simulink model "quadrupedRobot"  (R2020a)
settings: Solver=ode23tb  StartTime=0.0  StopTime=10  RelTol=1e-3
values from neighbouring files (symbols this model uses):
  BodyCenter_To_Arm = BodyLength*0.4    (= 0.24)    [Initial.m]
  BodyLength = 0.6    [Initial.m]
  BodyThick = 0.05    [Initial.m]
  BodyWidth = 0.25    [Initial.m]
  L1 = 0.1*L_total    (= 0.05)    [Initial.m]
  L2 = 0.4*L_total    (= 0.2)    [Initial.m]
  L3 = 0.5*L_total    (= 0.25)    [Initial.m]
  L_total = 0.5    [Initial.m]
  legX = 0.05    [Initial.m]
  legY = 0.05    [Initial.m]
  legZ = 0.05    [Initial.m]
  Mark = 1    [Initial.m]
  X = R_foot*cosd(0:0.2:90)    [Initial.m]
  X_FOOT = ([x_swing x_stance])/1000-S/2/2/1000    [Initial.m]
  Y = R_foot*sind(0:0.2:90)    [Initial.m]
  Y_FOOT = L1    (= 0.05)    [Initial.m]
  Z_FOOT = -L2-L3+Z_trajectory/1000+0.15    [Initial.m]
undefined symbols (not defined in the file or in its folder): Z
libraries: sm_lib x84, nesl_utility x27, Contact_Forces_Lib x5, simulink x1
(part 3 of 4)

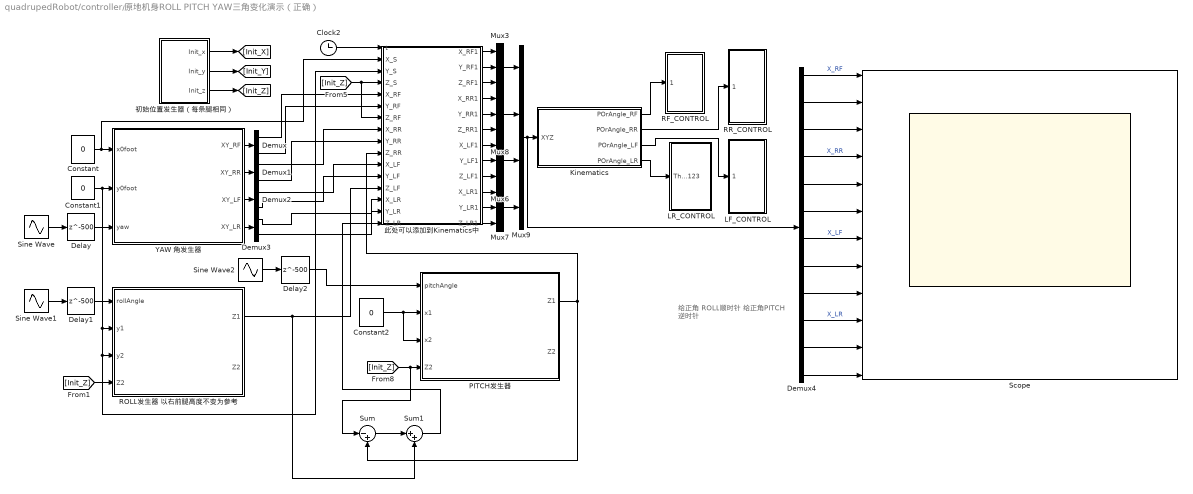
== system quadrupedRobot/controller/原地机身ROLL PITCH YAW三角变化演示（正确） ==
  note: 给正角 ROLL顺时针
      | 给正角PITCH 逆时针
  Clock2 : Clock
  Constant : Constant  Value=0
  Constant1 : Constant  Value=0
  Constant2 : Constant  Value=0
  Delay : Delay  DelayLength=500
  Delay1 : Delay  DelayLength=500
  Delay2 : Delay  DelayLength=500
  Demux{,1..3} (4 alike) : Demux  Outputs=2
  Demux4 : Demux  Outputs=12
  Kinematics : MATLAB Function  TreatAsAtomicUnit=on  mask{L1=L1, L2=L2, L3=L3, Mark=Mark}
  LF_CONTROL : Subsystem
  LR_CONTROL : Subsystem
  Mux{3,6..8} (4 alike) : Mux  Inputs=3
  Mux9 : Mux
  PITCH发生器 : MATLAB Function  TreatAsAtomicUnit=on
  RF_CONTROL : Subsystem
  ROLL发生器 以右前腿高度不变为参考 : MATLAB Function  TreatAsAtomicUnit=on
  RR_CONTROL : Subsystem
  Scope : Scope  NumInputPorts=12
  Sine Wave : Sin  Amplitude=8  Frequency=pi  SampleTime=0.001
  Sine Wave1 : Sin  Amplitude=8  Frequency=pi  SampleTime=0.001
  Sine Wave2 : Sin  Amplitude=8  Frequency=pi  SampleTime=0.001
  Sum : Sum  Inputs=|-+
  Sum1 : Sum  Inputs=|++
  YAW 角发生器 : MATLAB Function  TreatAsAtomicUnit=on
  初始位置发生器（每条腿相同） : Subsystem
  此处可以添加到Kinematics中 : Stateflow chart  TreatAsAtomicUnit=on
      settings: PortSchema="{\"entries\":[{\"content\":{\"sides\":[{\"content\":{\"connectorIds\":[\"In1\",\"In2\",\"In3\",\"In4\",\"In5\",\"In6\",\"In7\",\"In8\",\"In10\",\"In9\",\"In13\",\"In11\",\"In12\",\"In14\",\"In16\",\"In15\"]},\"type\":\"ConnectorPlacement.EquallySpacedRectSide\",\"uuid\":\"7e0be487-f0c2-4d3b-b1b4-d322333b651b\"},{\"content\":{\"connectorIds\":[\"Out11\",\"Out10\",\"Out9\",\"Out8\",\"Out6\",\"Out7\",\"Out3\",\"Out5\",\"Out4\",\"Out2\",\"Out12\",\"Out1\"],\"side\":\"RIGHT\"},\"type\":\"ConnectorPlacement.EquallySpacedRectSide\",\"uuid\":\"6febfd21-5bc4-4276-a755-f652306f84c9\"},{\"content\":{\"connectorIds\":[],\"side\":\"TOP\"},\"type\":\"ConnectorPlacement.EquallySpacedRectSide\",\"uuid\":\"b76ed853-f51f-41fe-9baf-83456c98e48b\"}]},\"type\":\"ConnectorPlacement.EquallySpacedConnector\",\"uuid\":\"3d522894-fd20-4e97-8ed2-383d7ec977f7\"}],\"packageUris\":[\"http://schema.mathworks.com/mf0/Connector/19700101\"],\"version\":\"1.0\"}"
  wires:
  Delay/1 -> YAW 角发生器/3(yaw)
  Demux3/2 -> 此处可以添加到Kinematics中/16(Y_LR)
  Demux3/1 -> 此处可以添加到Kinematics中/14(X_LR)
  YAW 角发生器/4(XY_LR) -> Demux3/1
  Demux2/2 -> 此处可以添加到Kinematics中/11(Y_LF)
  Demux2/1 -> 此处可以添加到Kinematics中/13(X_LF)
  YAW 角发生器/3(XY_LF) -> Demux2/1
  Demux1/1 -> 此处可以添加到Kinematics中/8(X_RR)
  YAW 角发生器/2(XY_RR) -> Demux1/1
  Demux/2 -> 此处可以添加到Kinematics中/6(Y_RF)
  Demux/1 -> 此处可以添加到Kinematics中/5(X_RF)
  YAW 角发生器/1(XY_RF) -> Demux/1
  Sine Wave/1 -> Delay/1
  初始位置发生器（每条腿相同）/1(Init_x) -> [Init_X]
  初始位置发生器（每条腿相同）/2(Init_y) -> [Init_Y]
  初始位置发生器（每条腿相同）/3(Init_z) -> [Init_Z]
  Constant/1 -> 此处可以添加到Kinematics中/2(X_S), YAW 角发生器/1(x0foot)
  [Init_Z] -> 此处可以添加到Kinematics中/7(Z_RF), 此处可以添加到Kinematics中/4(Z_S)
  Clock2/1 -> 此处可以添加到Kinematics中/1(t)
  此处可以添加到Kinematics中/11(X_RF1) -> Mux3/1
  此处可以添加到Kinematics中/10(Y_RF1) -> Mux3/2
  此处可以添加到Kinematics中/9(Z_RF1) -> Mux3/3
  此处可以添加到Kinematics中/8(X_RR1) -> Mux8/1
  此处可以添加到Kinematics中/6(Y_RR1) -> Mux8/2
  此处可以添加到Kinematics中/7(Z_RR1) -> Mux8/3
  此处可以添加到Kinematics中/3(X_LF1) -> Mux6/1
  此处可以添加到Kinematics中/5(Y_LF1) -> Mux6/2
  此处可以添加到Kinematics中/4(Z_LF1) -> Mux6/3
  此处可以添加到Kinematics中/2(X_LR1) -> Mux7/1
  此处可以添加到Kinematics中/12(Y_LR1) -> Mux7/2
  此处可以添加到Kinematics中/1(Z_LR1) -> Mux7/3
  Mux3/1 -> Mux9/1
  Mux8/1 -> Mux9/2
  Mux6/1 -> Mux9/3
  Mux7/1 -> Mux9/4
  Mux9/1 -> Demux4/1, Kinematics/1(XYZ)
  Kinematics/1(POrAngle_RF) -> RF_CONTROL/1(Theta123)
  Kinematics/2(POrAngle_RR) -> RR_CONTROL/1(Theta123)
  Kinematics/3(POrAngle_LF) -> LF_CONTROL/1(Theta123)
  Kinematics/4(POrAngle_LR) -> LR_CONTROL/1(Theta123)
  Sine Wave1/1 -> Delay1/1
  Delay1/1 -> ROLL发生器 以右前腿高度不变为参考/1(rollAngle)
  [Init_Z] -> ROLL发生器 以右前腿高度不变为参考/4("Z2 ")
  Constant1/1 -> ROLL发生器 以右前腿高度不变为参考/3(y2), 此处可以添加到Kinematics中/3(Y_S), ROLL发生器 以右前腿高度不变为参考/2(y1), YAW 角发生器/2(y0foot)
  ROLL发生器 以右前腿高度不变为参考/1(Z1) -> Sum1/2, 此处可以添加到Kinematics中/12(Z_LF)
  Constant2/1 -> PITCH发生器/2(x1), PITCH发生器/3(x2)
  PITCH发生器/1(Z1) -> Sum/2, 此处可以添加到Kinematics中/9(Z_RR)
  Sum/1 -> Sum1/1
  [Init_Z] -> Sum/1, PITCH发生器/4("Z2 ")
  Sum1/1 -> 此处可以添加到Kinematics中/15(Z_LR)
  Sine Wave2/1 -> Delay2/1
  Delay2/1 -> PITCH发生器/1(pitchAngle)
  Demux1/2 -> 此处可以添加到Kinematics中/10(Y_RR)
  Demux4/1 -> Scope/1  "X_RF"
  Demux4/2 -> Scope/2
  Demux4/3 -> Scope/3
  Demux4/4 -> Scope/4  "X_RR"
  Demux4/5 -> Scope/5
  Demux4/6 -> Scope/6
  Demux4/7 -> Scope/7  "X_LF"
  Demux4/8 -> Scope/8
  Demux4/9 -> Scope/9
  Demux4/10 -> Scope/10  "X_LR"
  Demux4/11 -> Scope/11
  Demux4/12 -> Scope/12

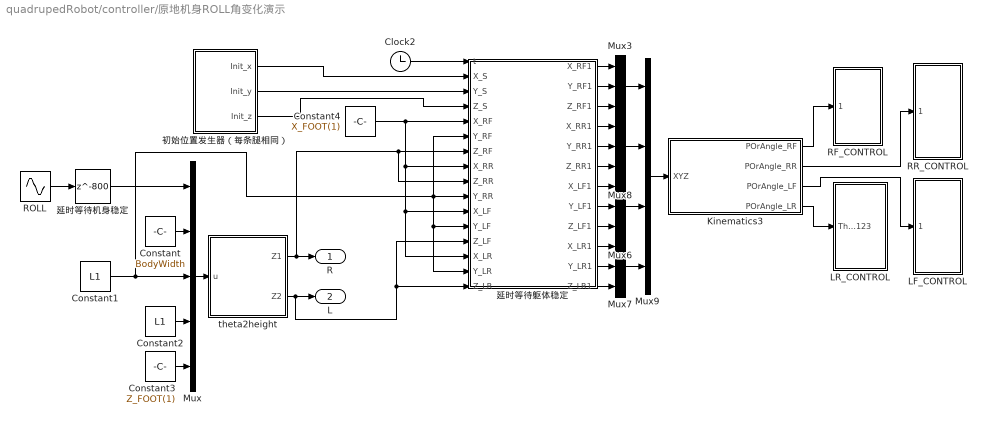
== system quadrupedRobot/controller/原地机身ROLL角变化演示 ==
  Clock2 : Clock
  Constant : Constant  Value=BodyWidth
  Constant1 : Constant  Value=L1
  Constant2 : Constant  Value=L1
  Constant3 : Constant  Value=Z_FOOT(1)
  Constant4 : Constant  Value=X_FOOT(1)
  Kinematics3 : MATLAB Function  TreatAsAtomicUnit=on  mask{L1=L1, L2=L2, L3=L3, Mark=Mark}
  LF_CONTROL : Subsystem
  LR_CONTROL : Subsystem
  Mux : Mux  Inputs=5
  Mux{3,6..8} (4 alike) : Mux  Inputs=3
  Mux9 : Mux
  RF_CONTROL : Subsystem
  ROLL : Sin  Amplitude=5  Frequency=3*pi  SampleTime=0.001
  RR_CONTROL : Subsystem
  theta2height : MATLAB Function  TreatAsAtomicUnit=on
  初始位置发生器（每条腿相同） : Subsystem
  延时等待机身稳定 : Delay  DelayLength=800
  延时等待躯体稳定 : Stateflow chart  TreatAsAtomicUnit=on
      settings: PortSchema="{\"entries\":[{\"content\":{\"sides\":[{\"content\":{\"connectorIds\":[\"In1\",\"In2\",\"In3\",\"In4\",\"In5\",\"In6\",\"In7\",\"In8\",\"In9\",\"In10\",\"In13\",\"In11\",\"In12\",\"In14\",\"In16\",\"In15\"]},\"type\":\"ConnectorPlacement.EquallySpacedRectSide\",\"uuid\":\"7e0be487-f0c2-4d3b-b1b4-d322333b651b\"},{\"content\":{\"connectorIds\":[\"Out11\",\"Out10\",\"Out9\",\"Out8\",\"Out6\",\"Out7\",\"Out3\",\"Out5\",\"Out4\",\"Out2\",\"Out12\",\"Out1\"],\"side\":\"RIGHT\"},\"type\":\"ConnectorPlacement.EquallySpacedRectSide\",\"uuid\":\"6febfd21-5bc4-4276-a755-f652306f84c9\"},{\"content\":{\"connectorIds\":[],\"side\":\"TOP\"},\"type\":\"ConnectorPlacement.EquallySpacedRectSide\",\"uuid\":\"b76ed853-f51f-41fe-9baf-83456c98e48b\"}]},\"type\":\"ConnectorPlacement.EquallySpacedConnector\",\"uuid\":\"3d522894-fd20-4e97-8ed2-383d7ec977f7\"}],\"packageUris\":[\"http://schema.mathworks.com/mf0/Connector/19700101\"],\"version\":\"1.0\"}"
  R : Outport
  L : Outport  Port=2
  wires:
  theta2height/2(Z2) -> 延时等待躯体稳定/12(Z_LF), 延时等待躯体稳定/15(Z_LR), L/1
  Mux/1 -> theta2height/1(u)
  ROLL/1 -> 延时等待机身稳定/1
  theta2height/1(Z1) -> 延时等待躯体稳定/9(Z_RR), 延时等待躯体稳定/7(Z_RF), R/1
  Kinematics3/3(POrAngle_LF) -> LF_CONTROL/1(Theta123)
  Kinematics3/2(POrAngle_RR) -> RR_CONTROL/1(Theta123)
  Mux8/1 -> Mux9/2
  延时等待躯体稳定/5(Y_LF1) -> Mux6/2
  Mux9/1 -> Kinematics3/1(XYZ)
  延时等待躯体稳定/1(Z_LR1) -> Mux7/3
  延时等待躯体稳定/11(X_RF1) -> Mux3/1
  延时等待躯体稳定/3(X_LF1) -> Mux6/1
  延时等待躯体稳定/6(Y_RR1) -> Mux8/2
  延时等待躯体稳定/2(X_LR1) -> Mux7/1
  延时等待躯体稳定/10(Y_RF1) -> Mux3/2
  延时等待躯体稳定/12(Y_LR1) -> Mux7/2
  Mux3/1 -> Mux9/1
  延时等待躯体稳定/9(Z_RF1) -> Mux3/3
  延时等待躯体稳定/7(Z_RR1) -> Mux8/3
  延时等待躯体稳定/4(Z_LF1) -> Mux6/3
  Kinematics3/1(POrAngle_RF) -> RF_CONTROL/1(Theta123)
  延时等待躯体稳定/8(X_RR1) -> Mux8/1
  初始位置发生器（每条腿相同）/2(Init_y) -> 延时等待躯体稳定/3(Y_S)
  Mux6/1 -> Mux9/3
  初始位置发生器（每条腿相同）/3(Init_z) -> 延时等待躯体稳定/4(Z_S)
  Clock2/1 -> 延时等待躯体稳定/1(t)
  Mux7/1 -> Mux9/4
  Kinematics3/4(POrAngle_LR) -> LR_CONTROL/1(Theta123)
  初始位置发生器（每条腿相同）/1(Init_x) -> 延时等待躯体稳定/2(X_S)
  Constant/1 -> Mux/2
  Constant1/1 -> Mux/3, 延时等待躯体稳定/6(Y_RF), 延时等待躯体稳定/11(Y_LF), 延时等待躯体稳定/16(Y_LR), 延时等待躯体稳定/10(Y_RR)
  Constant2/1 -> Mux/4
  Constant3/1 -> Mux/5
  Constant4/1 -> 延时等待躯体稳定/14(X_LR), 延时等待躯体稳定/13(X_LF), 延时等待躯体稳定/8(X_RR), 延时等待躯体稳定/5(X_RF)
  延时等待机身稳定/1 -> Mux/1

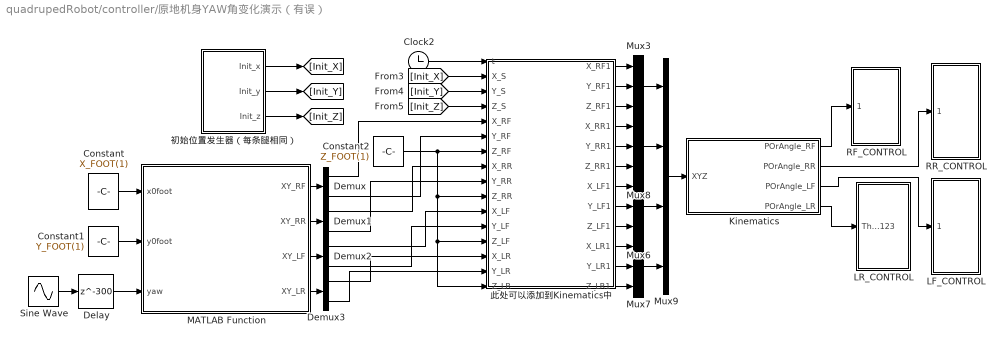
== system quadrupedRobot/controller/原地机身YAW角变化演示（有误） ==
  Clock2 : Clock
  Constant : Constant  Value=X_FOOT(1)
  Constant1 : Constant  Value=Y_FOOT(1)
  Constant2 : Constant  Value=Z_FOOT(1)
  Delay : Delay  DelayLength=300
  Demux{,1..3} (4 alike) : Demux  Outputs=2
  Kinematics : MATLAB Function  TreatAsAtomicUnit=on  mask{L1=L1, L2=L2, L3=L3, Mark=Mark}
  LF_CONTROL : Subsystem
  LR_CONTROL : Subsystem
  MATLAB Function : MATLAB Function  TreatAsAtomicUnit=on
  Mux{3,6..8} (4 alike) : Mux  Inputs=3
  Mux9 : Mux
  RF_CONTROL : Subsystem
  RR_CONTROL : Subsystem
  Sine Wave : Sin  Amplitude=10  Frequency=2*pi  SampleTime=0.001
  初始位置发生器（每条腿相同） : Subsystem
  此处可以添加到Kinematics中 : Stateflow chart  TreatAsAtomicUnit=on
      settings: PortSchema="{\"entries\":[{\"content\":{\"sides\":[{\"content\":{\"connectorIds\":[\"In1\",\"In2\",\"In3\",\"In4\",\"In5\",\"In6\",\"In7\",\"In8\",\"In10\",\"In9\",\"In13\",\"In11\",\"In12\",\"In14\",\"In16\",\"In15\"]},\"type\":\"ConnectorPlacement.EquallySpacedRectSide\",\"uuid\":\"7e0be487-f0c2-4d3b-b1b4-d322333b651b\"},{\"content\":{\"connectorIds\":[\"Out11\",\"Out10\",\"Out9\",\"Out8\",\"Out6\",\"Out7\",\"Out3\",\"Out5\",\"Out4\",\"Out2\",\"Out12\",\"Out1\"],\"side\":\"RIGHT\"},\"type\":\"ConnectorPlacement.EquallySpacedRectSide\",\"uuid\":\"6febfd21-5bc4-4276-a755-f652306f84c9\"},{\"content\":{\"connectorIds\":[],\"side\":\"TOP\"},\"type\":\"ConnectorPlacement.EquallySpacedRectSide\",\"uuid\":\"b76ed853-f51f-41fe-9baf-83456c98e48b\"}]},\"type\":\"ConnectorPlacement.EquallySpacedConnector\",\"uuid\":\"3d522894-fd20-4e97-8ed2-383d7ec977f7\"}],\"packageUris\":[\"http://schema.mathworks.com/mf0/Connector/19700101\"],\"version\":\"1.0\"}"
  wires:
  Kinematics/4(POrAngle_LR) -> LR_CONTROL/1(Theta123)
  Kinematics/3(POrAngle_LF) -> LF_CONTROL/1(Theta123)
  Kinematics/2(POrAngle_RR) -> RR_CONTROL/1(Theta123)
  Kinematics/1(POrAngle_RF) -> RF_CONTROL/1(Theta123)
  Mux9/1 -> Kinematics/1(XYZ)
  Mux7/1 -> Mux9/4
  Mux6/1 -> Mux9/3
  Mux8/1 -> Mux9/2
  Mux3/1 -> Mux9/1
  此处可以添加到Kinematics中/1(Z_LR1) -> Mux7/3
  此处可以添加到Kinematics中/12(Y_LR1) -> Mux7/2
  此处可以添加到Kinematics中/2(X_LR1) -> Mux7/1
  此处可以添加到Kinematics中/4(Z_LF1) -> Mux6/3
  此处可以添加到Kinematics中/5(Y_LF1) -> Mux6/2
  此处可以添加到Kinematics中/3(X_LF1) -> Mux6/1
  此处可以添加到Kinematics中/7(Z_RR1) -> Mux8/3
  此处可以添加到Kinematics中/6(Y_RR1) -> Mux8/2
  此处可以添加到Kinematics中/8(X_RR1) -> Mux8/1
  此处可以添加到Kinematics中/9(Z_RF1) -> Mux3/3
  此处可以添加到Kinematics中/10(Y_RF1) -> Mux3/2
  此处可以添加到Kinematics中/11(X_RF1) -> Mux3/1
  Clock2/1 -> 此处可以添加到Kinematics中/1(t)
  [Init_Z] -> 此处可以添加到Kinematics中/4(Z_S)
  [Init_Y] -> 此处可以添加到Kinematics中/3(Y_S)
  [Init_X] -> 此处可以添加到Kinematics中/2(X_S)
  初始位置发生器（每条腿相同）/3(Init_z) -> [Init_Z]
  初始位置发生器（每条腿相同）/2(Init_y) -> [Init_Y]
  初始位置发生器（每条腿相同）/1(Init_x) -> [Init_X]
  ? -> ?
  Constant/1 -> MATLAB Function/1(x0foot)
  Constant1/1 -> MATLAB Function/2(y0foot)
  Sine Wave/1 -> Delay/1
  Constant2/1 -> 此处可以添加到Kinematics中/15(Z_LR), 此处可以添加到Kinematics中/12(Z_LF), 此处可以添加到Kinematics中/9(Z_RR), 此处可以添加到Kinematics中/7(Z_RF)
  MATLAB Function/1(XY_RF) -> Demux/1
  Demux/1 -> 此处可以添加到Kinematics中/5(X_RF)
  Demux/2 -> 此处可以添加到Kinematics中/6(Y_RF)
  MATLAB Function/2(XY_RR) -> Demux1/1
  Demux1/1 -> 此处可以添加到Kinematics中/8(X_RR)
  Demux1/2 -> 此处可以添加到Kinematics中/10(Y_RR)
  MATLAB Function/3(XY_LF) -> Demux2/1
  Demux2/1 -> 此处可以添加到Kinematics中/13(X_LF)
  Demux2/2 -> 此处可以添加到Kinematics中/11(Y_LF)
  MATLAB Function/4(XY_LR) -> Demux3/1
  Demux3/1 -> 此处可以添加到Kinematics中/14(X_LR)
  Demux3/2 -> 此处可以添加到Kinematics中/16(Y_LR)
  Delay/1 -> MATLAB Function/3(yaw)

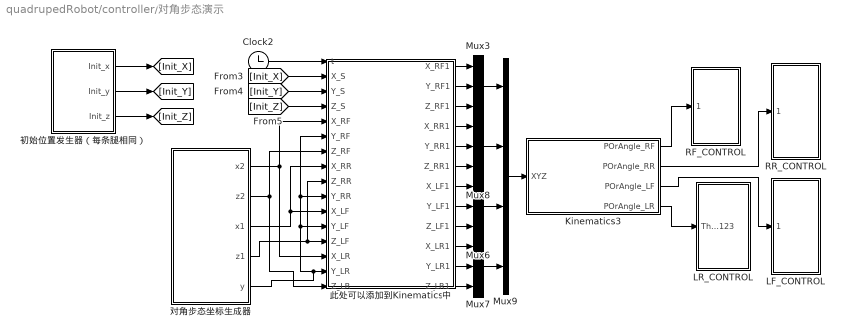
== system quadrupedRobot/controller/对角步态演示 ==
  Clock2 : Clock
  Kinematics3 : MATLAB Function  TreatAsAtomicUnit=on  mask{L1=L1, L2=L2, L3=L3, Mark=Mark}
  LF_CONTROL : Subsystem
  LR_CONTROL : Subsystem
  Mux{3,6..8} (4 alike) : Mux  Inputs=3
  Mux9 : Mux
  RF_CONTROL : Subsystem
  RR_CONTROL : Subsystem
  初始位置发生器（每条腿相同） : Subsystem
  对角步态坐标生成器 : Subsystem
  此处可以添加到Kinematics中 : Stateflow chart  TreatAsAtomicUnit=on
      settings: PortSchema="{\"entries\":[{\"content\":{\"sides\":[{\"content\":{\"connectorIds\":[\"In1\",\"In2\",\"In3\",\"In4\",\"In5\",\"In6\",\"In7\",\"In8\",\"In9\",\"In10\",\"In13\",\"In11\",\"In12\",\"In14\",\"In16\",\"In15\"]},\"type\":\"ConnectorPlacement.EquallySpacedRectSide\",\"uuid\":\"7e0be487-f0c2-4d3b-b1b4-d322333b651b\"},{\"content\":{\"connectorIds\":[\"Out11\",\"Out10\",\"Out9\",\"Out8\",\"Out6\",\"Out7\",\"Out3\",\"Out5\",\"Out4\",\"Out2\",\"Out12\",\"Out1\"],\"side\":\"RIGHT\"},\"type\":\"ConnectorPlacement.EquallySpacedRectSide\",\"uuid\":\"6febfd21-5bc4-4276-a755-f652306f84c9\"},{\"content\":{\"connectorIds\":[],\"side\":\"TOP\"},\"type\":\"ConnectorPlacement.EquallySpacedRectSide\",\"uuid\":\"b76ed853-f51f-41fe-9baf-83456c98e48b\"}]},\"type\":\"ConnectorPlacement.EquallySpacedConnector\",\"uuid\":\"3d522894-fd20-4e97-8ed2-383d7ec977f7\"}],\"packageUris\":[\"http://schema.mathworks.com/mf0/Connector/19700101\"],\"version\":\"1.0\"}"
  wires:
  ? -> ?
  初始位置发生器（每条腿相同）/1(Init_x) -> [Init_X]
  初始位置发生器（每条腿相同）/2(Init_y) -> [Init_Y]
  初始位置发生器（每条腿相同）/3(Init_z) -> [Init_Z]
  [Init_X] -> 此处可以添加到Kinematics中/2(X_S)
  [Init_Y] -> 此处可以添加到Kinematics中/3(Y_S)
  [Init_Z] -> 此处可以添加到Kinematics中/4(Z_S)
  Clock2/1 -> 此处可以添加到Kinematics中/1(t)
  此处可以添加到Kinematics中/11(X_RF1) -> Mux3/1
  此处可以添加到Kinematics中/10(Y_RF1) -> Mux3/2
  此处可以添加到Kinematics中/9(Z_RF1) -> Mux3/3
  此处可以添加到Kinematics中/8(X_RR1) -> Mux8/1
  此处可以添加到Kinematics中/6(Y_RR1) -> Mux8/2
  此处可以添加到Kinematics中/7(Z_RR1) -> Mux8/3
  此处可以添加到Kinematics中/3(X_LF1) -> Mux6/1
  此处可以添加到Kinematics中/5(Y_LF1) -> Mux6/2
  此处可以添加到Kinematics中/4(Z_LF1) -> Mux6/3
  此处可以添加到Kinematics中/2(X_LR1) -> Mux7/1
  此处可以添加到Kinematics中/12(Y_LR1) -> Mux7/2
  此处可以添加到Kinematics中/1(Z_LR1) -> Mux7/3
  Mux3/1 -> Mux9/1
  Mux8/1 -> Mux9/2
  Mux6/1 -> Mux9/3
  Mux7/1 -> Mux9/4
  Mux9/1 -> Kinematics3/1(XYZ)
  Kinematics3/1(POrAngle_RF) -> RF_CONTROL/1(Theta123)
  Kinematics3/2(POrAngle_RR) -> RR_CONTROL/1(Theta123)
  Kinematics3/3(POrAngle_LF) -> LF_CONTROL/1(Theta123)
  Kinematics3/4(POrAngle_LR) -> LR_CONTROL/1(Theta123)
  对角步态坐标生成器/5(y) -> 此处可以添加到Kinematics中/11(Y_LF), 此处可以添加到Kinematics中/6(Y_RF), 此处可以添加到Kinematics中/10(Y_RR), 此处可以添加到Kinematics中/16(Y_LR)
  对角步态坐标生成器/1(x2) -> 此处可以添加到Kinematics中/14(X_LR), 此处可以添加到Kinematics中/5(X_RF)
  对角步态坐标生成器/2(z2) -> 此处可以添加到Kinematics中/7(Z_RF), 此处可以添加到Kinematics中/15(Z_LR)
  对角步态坐标生成器/3(x1) -> 此处可以添加到Kinematics中/13(X_LF), 此处可以添加到Kinematics中/8(X_RR)
  对角步态坐标生成器/4(z1) -> 此处可以添加到Kinematics中/9(Z_RR), 此处可以添加到Kinematics中/12(Z_LF)

== system quadrupedRobot/Robot/LF/Subsystem ==
  shoulderJoint : Inport
  R1 : sm_lib/Joints/Revolute Joint  JointMode=Normal  SenseConstraintForce=off  SenseConstraintForceX=off  SenseConstraintForceY=off  SenseConstraintForceZ=off  SenseConstraintTorque=off  SenseConstraintTorqueX=off  SenseConstraintTorqueY=off  SenseConstraintTorqueZ=off  SenseTotalForce=off  SenseTotalForceX=off  SenseTotalForceY=off  SenseTotalForceZ=off  SenseTotalTorque=off  SenseTotalTorqueX=off  SenseTotalTorqueY=off  SenseTotalTorqueZ=off  CompositeWrenchDir=FollowerOnBase  CompositeWrenchFrame=BaseFrame  EquilibriumPosition=0  EquilibriumPositionUnits=deg  SpringStiffness=0  SpringStiffnessUnits=N*m/deg  DampingCoefficient=0  DampingCoefficientUnits=N*m/(deg/s)  TorqueActuationMode=ComputedTorque  MotionActuationMode=InputMotion  SensePosition=off  SenseVelocity=off  SenseAcceleration=off  SenseTorqueForce=off  SenseLowerLimitTorqueForce=off  SenseUpperLimitTorqueForce=off  LowerLimitSpecify=off  LowerLimitBound=-90  LowerLimitBoundUnits=deg  LowerLimitStiffness=1e4  LowerLimitStiffnessUnits=N*m/deg  LowerLimitDamping=10  LowerLimitDampingUnits=N*m/(deg/s)  LowerLimitTransitionRegionWidth=0.1  LowerLimitTransitionRegionWidthUnits=deg  UpperLimitSpecify=off  UpperLimitBound=90  UpperLimitBoundUnits=deg  UpperLimitStiffness=1e4  UpperLimitStiffnessUnits=N*m/deg  UpperLimitDamping=10  UpperLimitDampingUnits=N*m/(deg/s)  UpperLimitTransitionRegionWidth=0.1  UpperLimitTransitionRegionWidthUnits=deg  PositionTargetSpecify=on  PositionTargetPriority=High  PositionTargetValue=0  PositionTargetValueUnits=deg  VelocityTargetSpecify=off  VelocityTargetPriority=High  VelocityTargetValue=0  VelocityTargetValueUnits=deg/s
  Rigid Transform8 : sm_lib/Frames and Transforms/Rigid Transform  TranslationMethod=None  TranslationStandardOffset=0  TranslationLengthUnit=m  TranslationStandardAxis=+Z  TranslationCartesianOffset=[0 0 0]  TranslationROffset=0  TranslationROffsetUnits=m  TranslationZOffset=0  TranslationZOffsetUnits=m  TranslationThetaOffset=0  TranslationThetaOffsetUnits=deg  RotationMethod=StandardAxis  RotationAngleUnits=deg  RotationStandardAxis=+Y  RotationAngle=90  RotationArbitraryAxis=[0 0 1]  FollAlignAxisA=+X  BaseAlignAxisA=+Y  FollAlignAxisB=+Y  BaseAlignAxisB=+Z  RotationSequenceAxes=FollowerAxes  RotationSequence=XYX  RotationSequenceAngles=[0 0 0]  RotationSequenceAnglesUnits=deg  RotationMatrix=[1 0 0; 0 1 0; 0 0 1]
  Rigid Transform9 : sm_lib/Frames and Transforms/Rigid Transform  TranslationMethod=None  TranslationStandardOffset=0  TranslationLengthUnit=m  TranslationStandardAxis=+Z  TranslationCartesianOffset=[0 0 0]  TranslationROffset=0  TranslationROffsetUnits=m  TranslationZOffset=0  TranslationZOffsetUnits=m  TranslationThetaOffset=0  TranslationThetaOffsetUnits=deg  RotationMethod=StandardAxis  RotationAngleUnits=deg  RotationStandardAxis=+Y  RotationAngle=90  RotationArbitraryAxis=[0 0 1]  FollAlignAxisA=+X  BaseAlignAxisA=+Y  FollAlignAxisB=+Y  BaseAlignAxisB=+Z  RotationSequenceAxes=FollowerAxes  RotationSequence=XYX  RotationSequenceAngles=[0 0 0]  RotationSequenceAnglesUnits=deg  RotationMatrix=[1 0 0; 0 1 0; 0 0 1]
  Simulink-PS Converter4 : nesl_utility/Simulink-PS Converter  PhysicalDomain=network_engine_domain  SubClassName=ps_input  LeftPortType=input  RightPortType=output  PseudoPeriodic=off  Frequencies=[]  NoiseDistribution=none  NoiseParameters=[]  Unit=1  AffineConversion=off  FilteringAndDerivatives=filter  SimscapeFilterOrder=2  InputFilterTimeConstant=0.001  UdotUserProvided=0
  B1 : PMIOPort  Side=Left
  B2 : PMIOPort  Port=2  Side=Right
  wires:
  shoulderJoint/1 -> Simulink-PS Converter4/1
  connections:
  Rigid Transform9/LConn1 -- B2/RConn1
  Rigid Transform8/LConn1 -- B1/RConn1
  R1/RConn1 -- Rigid Transform9/RConn1
  Simulink-PS Converter4/RConn1 -- R1/LConn2
  Rigid Transform8/RConn1 -- R1/LConn1

== system quadrupedRobot/Robot/LF/Subsystem1 ==
  upperJoint : Inport
  R2 : sm_lib/Joints/Revolute Joint  JointMode=Normal  SenseConstraintForce=off  SenseConstraintForceX=off  SenseConstraintForceY=off  SenseConstraintForceZ=off  SenseConstraintTorque=off  SenseConstraintTorqueX=off  SenseConstraintTorqueY=off  SenseConstraintTorqueZ=off  SenseTotalForce=off  SenseTotalForceX=off  SenseTotalForceY=off  SenseTotalForceZ=off  SenseTotalTorque=off  SenseTotalTorqueX=off  SenseTotalTorqueY=off  SenseTotalTorqueZ=off  CompositeWrenchDir=FollowerOnBase  CompositeWrenchFrame=BaseFrame  EquilibriumPosition=0  EquilibriumPositionUnits=deg  SpringStiffness=0  SpringStiffnessUnits=N*m/deg  DampingCoefficient=0  DampingCoefficientUnits=N*m/(deg/s)  TorqueActuationMode=ComputedTorque  MotionActuationMode=InputMotion  SensePosition=off  SenseVelocity=off  SenseAcceleration=off  SenseTorqueForce=off  SenseLowerLimitTorqueForce=off  SenseUpperLimitTorqueForce=off  LowerLimitSpecify=off  LowerLimitBound=-90  LowerLimitBoundUnits=deg  LowerLimitStiffness=1e4  LowerLimitStiffnessUnits=N*m/deg  LowerLimitDamping=10  LowerLimitDampingUnits=N*m/(deg/s)  LowerLimitTransitionRegionWidth=0.1  LowerLimitTransitionRegionWidthUnits=deg  UpperLimitSpecify=off  UpperLimitBound=90  UpperLimitBoundUnits=deg  UpperLimitStiffness=1e4  UpperLimitStiffnessUnits=N*m/deg  UpperLimitDamping=10  UpperLimitDampingUnits=N*m/(deg/s)  UpperLimitTransitionRegionWidth=0.1  UpperLimitTransitionRegionWidthUnits=deg  PositionTargetSpecify=on  PositionTargetPriority=High  PositionTargetValue=0  PositionTargetValueUnits=deg  VelocityTargetSpecify=off  VelocityTargetPriority=High  VelocityTargetValue=0  VelocityTargetValueUnits=deg/s
  Rigid Transform8 : sm_lib/Frames and Transforms/Rigid Transform  TranslationMethod=None  TranslationStandardOffset=0  TranslationLengthUnit=m  TranslationStandardAxis=+Z  TranslationCartesianOffset=[0 0 0]  TranslationROffset=0  TranslationROffsetUnits=m  TranslationZOffset=0  TranslationZOffsetUnits=m  TranslationThetaOffset=0  TranslationThetaOffsetUnits=deg  RotationMethod=StandardAxis  RotationAngleUnits=deg  RotationStandardAxis=+X  RotationAngle=90  RotationArbitraryAxis=[0 0 1]  FollAlignAxisA=+X  BaseAlignAxisA=+Y  FollAlignAxisB=+Y  BaseAlignAxisB=+Z  RotationSequenceAxes=FollowerAxes  RotationSequence=XYX  RotationSequenceAngles=[0 0 0]  RotationSequenceAnglesUnits=deg  RotationMatrix=[1 0 0; 0 1 0; 0 0 1]
  Rigid Transform9 : sm_lib/Frames and Transforms/Rigid Transform  TranslationMethod=None  TranslationStandardOffset=0  TranslationLengthUnit=m  TranslationStandardAxis=+Z  TranslationCartesianOffset=[0 0 0]  TranslationROffset=0  TranslationROffsetUnits=m  TranslationZOffset=0  TranslationZOffsetUnits=m  TranslationThetaOffset=0  TranslationThetaOffsetUnits=deg  RotationMethod=StandardAxis  RotationAngleUnits=deg  RotationStandardAxis=+X  RotationAngle=90  RotationArbitraryAxis=[0 0 1]  FollAlignAxisA=+X  BaseAlignAxisA=+Y  FollAlignAxisB=+Y  BaseAlignAxisB=+Z  RotationSequenceAxes=FollowerAxes  RotationSequence=XYX  RotationSequenceAngles=[0 0 0]  RotationSequenceAnglesUnits=deg  RotationMatrix=[1 0 0; 0 1 0; 0 0 1]
  Simulink-PS Converter4 : nesl_utility/Simulink-PS Converter  PhysicalDomain=network_engine_domain  SubClassName=ps_input  LeftPortType=input  RightPortType=output  PseudoPeriodic=off  Frequencies=[]  NoiseDistribution=none  NoiseParameters=[]  Unit=1  AffineConversion=off  FilteringAndDerivatives=filter  SimscapeFilterOrder=2  InputFilterTimeConstant=0.001  UdotUserProvided=0
  B1 : PMIOPort  Side=Left
  B2 : PMIOPort  Port=2  Side=Right
  wires:
  upperJoint/1 -> Simulink-PS Converter4/1
  connections:
  Simulink-PS Converter4/RConn1 -- R2/LConn2
  Rigid Transform8/RConn1 -- R2/LConn1
  R2/RConn1 -- Rigid Transform9/RConn1
  Rigid Transform8/LConn1 -- B1/RConn1
  Rigid Transform9/LConn1 -- B2/RConn1

== system quadrupedRobot/Robot/LF/Subsystem2 ==
  lowerJoint : Inport
  R3 : sm_lib/Joints/Revolute Joint  JointMode=Normal  SenseConstraintForce=off  SenseConstraintForceX=off  SenseConstraintForceY=off  SenseConstraintForceZ=off  SenseConstraintTorque=off  SenseConstraintTorqueX=off  SenseConstraintTorqueY=off  SenseConstraintTorqueZ=off  SenseTotalForce=off  SenseTotalForceX=off  SenseTotalForceY=off  SenseTotalForceZ=off  SenseTotalTorque=off  SenseTotalTorqueX=off  SenseTotalTorqueY=off  SenseTotalTorqueZ=off  CompositeWrenchDir=FollowerOnBase  CompositeWrenchFrame=BaseFrame  EquilibriumPosition=0  EquilibriumPositionUnits=deg  SpringStiffness=0  SpringStiffnessUnits=N*m/deg  DampingCoefficient=0  DampingCoefficientUnits=N*m/(deg/s)  TorqueActuationMode=ComputedTorque  MotionActuationMode=InputMotion  SensePosition=off  SenseVelocity=off  SenseAcceleration=off  SenseTorqueForce=off  SenseLowerLimitTorqueForce=off  SenseUpperLimitTorqueForce=off  LowerLimitSpecify=off  LowerLimitBound=-90  LowerLimitBoundUnits=deg  LowerLimitStiffness=1e4  LowerLimitStiffnessUnits=N*m/deg  LowerLimitDamping=10  LowerLimitDampingUnits=N*m/(deg/s)  LowerLimitTransitionRegionWidth=0.1  LowerLimitTransitionRegionWidthUnits=deg  UpperLimitSpecify=off  UpperLimitBound=90  UpperLimitBoundUnits=deg  UpperLimitStiffness=1e4  UpperLimitStiffnessUnits=N*m/deg  UpperLimitDamping=10  UpperLimitDampingUnits=N*m/(deg/s)  UpperLimitTransitionRegionWidth=0.1  UpperLimitTransitionRegionWidthUnits=deg  PositionTargetSpecify=on  PositionTargetPriority=High  PositionTargetValue=0  PositionTargetValueUnits=deg  VelocityTargetSpecify=off  VelocityTargetPriority=High  VelocityTargetValue=0  VelocityTargetValueUnits=deg/s
  Rigid Transform8 : sm_lib/Frames and Transforms/Rigid Transform  TranslationMethod=None  TranslationStandardOffset=0  TranslationLengthUnit=m  TranslationStandardAxis=+Z  TranslationCartesianOffset=[0 0 0]  TranslationROffset=0  TranslationROffsetUnits=m  TranslationZOffset=0  TranslationZOffsetUnits=m  TranslationThetaOffset=0  TranslationThetaOffsetUnits=deg  RotationMethod=StandardAxis  RotationAngleUnits=deg  RotationStandardAxis=+X  RotationAngle=90  RotationArbitraryAxis=[0 0 1]  FollAlignAxisA=+X  BaseAlignAxisA=+Y  FollAlignAxisB=+Y  BaseAlignAxisB=+Z  RotationSequenceAxes=FollowerAxes  RotationSequence=XYX  RotationSequenceAngles=[0 0 0]  RotationSequenceAnglesUnits=deg  RotationMatrix=[1 0 0; 0 1 0; 0 0 1]
  Rigid Transform9 : sm_lib/Frames and Transforms/Rigid Transform  TranslationMethod=None  TranslationStandardOffset=0  TranslationLengthUnit=m  TranslationStandardAxis=+Z  TranslationCartesianOffset=[0 0 0]  TranslationROffset=0  TranslationROffsetUnits=m  TranslationZOffset=0  TranslationZOffsetUnits=m  TranslationThetaOffset=0  TranslationThetaOffsetUnits=deg  RotationMethod=StandardAxis  RotationAngleUnits=deg  RotationStandardAxis=+X  RotationAngle=90  RotationArbitraryAxis=[0 0 1]  FollAlignAxisA=+X  BaseAlignAxisA=+Y  FollAlignAxisB=+Y  BaseAlignAxisB=+Z  RotationSequenceAxes=FollowerAxes  RotationSequence=XYX  RotationSequenceAngles=[0 0 0]  RotationSequenceAnglesUnits=deg  RotationMatrix=[1 0 0; 0 1 0; 0 0 1]
  Simulink-PS Converter : nesl_utility/Simulink-PS Converter  PhysicalDomain=network_engine_domain  SubClassName=ps_input  LeftPortType=input  RightPortType=output  PseudoPeriodic=off  Frequencies=[]  NoiseDistribution=none  NoiseParameters=[]  Unit=1  AffineConversion=off  FilteringAndDerivatives=filter  SimscapeFilterOrder=2  InputFilterTimeConstant=0.001  UdotUserProvided=0
  B1 : PMIOPort  Side=Left
  B2 : PMIOPort  Port=2  Side=Right
  wires:
  lowerJoint/1 -> Simulink-PS Converter/1
  connections:
  Rigid Transform8/RConn1 -- R3/LConn1
  Simulink-PS Converter/RConn1 -- R3/LConn2
  R3/RConn1 -- Rigid Transform9/RConn1
  Rigid Transform8/LConn1 -- B1/RConn1
  Rigid Transform9/LConn1 -- B2/RConn1

== system quadrupedRobot/Robot/LR/Subsystem ==
  shoulderJoint : Inport
  R1 : sm_lib/Joints/Revolute Joint  JointMode=Normal  SenseConstraintForce=off  SenseConstraintForceX=off  SenseConstraintForceY=off  SenseConstraintForceZ=off  SenseConstraintTorque=off  SenseConstraintTorqueX=off  SenseConstraintTorqueY=off  SenseConstraintTorqueZ=off  SenseTotalForce=off  SenseTotalForceX=off  SenseTotalForceY=off  SenseTotalForceZ=off  SenseTotalTorque=off  SenseTotalTorqueX=off  SenseTotalTorqueY=off  SenseTotalTorqueZ=off  CompositeWrenchDir=FollowerOnBase  CompositeWrenchFrame=BaseFrame  EquilibriumPosition=0  EquilibriumPositionUnits=deg  SpringStiffness=0  SpringStiffnessUnits=N*m/deg  DampingCoefficient=0  DampingCoefficientUnits=N*m/(deg/s)  TorqueActuationMode=ComputedTorque  MotionActuationMode=InputMotion  SensePosition=off  SenseVelocity=off  SenseAcceleration=off  SenseTorqueForce=off  SenseLowerLimitTorqueForce=off  SenseUpperLimitTorqueForce=off  LowerLimitSpecify=off  LowerLimitBound=-90  LowerLimitBoundUnits=deg  LowerLimitStiffness=1e4  LowerLimitStiffnessUnits=N*m/deg  LowerLimitDamping=10  LowerLimitDampingUnits=N*m/(deg/s)  LowerLimitTransitionRegionWidth=0.1  LowerLimitTransitionRegionWidthUnits=deg  UpperLimitSpecify=off  UpperLimitBound=90  UpperLimitBoundUnits=deg  UpperLimitStiffness=1e4  UpperLimitStiffnessUnits=N*m/deg  UpperLimitDamping=10  UpperLimitDampingUnits=N*m/(deg/s)  UpperLimitTransitionRegionWidth=0.1  UpperLimitTransitionRegionWidthUnits=deg  PositionTargetSpecify=on  PositionTargetPriority=High  PositionTargetValue=0  PositionTargetValueUnits=deg  VelocityTargetSpecify=off  VelocityTargetPriority=High  VelocityTargetValue=0  VelocityTargetValueUnits=deg/s
  Rigid Transform8 : sm_lib/Frames and Transforms/Rigid Transform  TranslationMethod=None  TranslationStandardOffset=0  TranslationLengthUnit=m  TranslationStandardAxis=+Z  TranslationCartesianOffset=[0 0 0]  TranslationROffset=0  TranslationROffsetUnits=m  TranslationZOffset=0  TranslationZOffsetUnits=m  TranslationThetaOffset=0  TranslationThetaOffsetUnits=deg  RotationMethod=StandardAxis  RotationAngleUnits=deg  RotationStandardAxis=+Y  RotationAngle=90  RotationArbitraryAxis=[0 0 1]  FollAlignAxisA=+X  BaseAlignAxisA=+Y  FollAlignAxisB=+Y  BaseAlignAxisB=+Z  RotationSequenceAxes=FollowerAxes  RotationSequence=XYX  RotationSequenceAngles=[0 0 0]  RotationSequenceAnglesUnits=deg  RotationMatrix=[1 0 0; 0 1 0; 0 0 1]
  Rigid Transform9 : sm_lib/Frames and Transforms/Rigid Transform  TranslationMethod=None  TranslationStandardOffset=0  TranslationLengthUnit=m  TranslationStandardAxis=+Z  TranslationCartesianOffset=[0 0 0]  TranslationROffset=0  TranslationROffsetUnits=m  TranslationZOffset=0  TranslationZOffsetUnits=m  TranslationThetaOffset=0  TranslationThetaOffsetUnits=deg  RotationMethod=StandardAxis  RotationAngleUnits=deg  RotationStandardAxis=+Y  RotationAngle=90  RotationArbitraryAxis=[0 0 1]  FollAlignAxisA=+X  BaseAlignAxisA=+Y  FollAlignAxisB=+Y  BaseAlignAxisB=+Z  RotationSequenceAxes=FollowerAxes  RotationSequence=XYX  RotationSequenceAngles=[0 0 0]  RotationSequenceAnglesUnits=deg  RotationMatrix=[1 0 0; 0 1 0; 0 0 1]
  Simulink-PS Converter4 : nesl_utility/Simulink-PS Converter  PhysicalDomain=network_engine_domain  SubClassName=ps_input  LeftPortType=input  RightPortType=output  PseudoPeriodic=off  Frequencies=[]  NoiseDistribution=none  NoiseParameters=[]  Unit=1  AffineConversion=off  FilteringAndDerivatives=filter  SimscapeFilterOrder=2  InputFilterTimeConstant=0.001  UdotUserProvided=0
  B1 : PMIOPort  Side=Left
  B2 : PMIOPort  Port=2  Side=Right
  wires:
  shoulderJoint/1 -> Simulink-PS Converter4/1
  connections:
  Rigid Transform8/RConn1 -- R1/LConn1
  Simulink-PS Converter4/RConn1 -- R1/LConn2
  R1/RConn1 -- Rigid Transform9/RConn1
  Rigid Transform8/LConn1 -- B1/RConn1
  Rigid Transform9/LConn1 -- B2/RConn1

== system quadrupedRobot/Robot/LR/Subsystem1 ==
  upperJoint : Inport
  R2 : sm_lib/Joints/Revolute Joint  JointMode=Normal  SenseConstraintForce=off  SenseConstraintForceX=off  SenseConstraintForceY=off  SenseConstraintForceZ=off  SenseConstraintTorque=off  SenseConstraintTorqueX=off  SenseConstraintTorqueY=off  SenseConstraintTorqueZ=off  SenseTotalForce=off  SenseTotalForceX=off  SenseTotalForceY=off  SenseTotalForceZ=off  SenseTotalTorque=off  SenseTotalTorqueX=off  SenseTotalTorqueY=off  SenseTotalTorqueZ=off  CompositeWrenchDir=FollowerOnBase  CompositeWrenchFrame=BaseFrame  EquilibriumPosition=0  EquilibriumPositionUnits=deg  SpringStiffness=0  SpringStiffnessUnits=N*m/deg  DampingCoefficient=0  DampingCoefficientUnits=N*m/(deg/s)  TorqueActuationMode=ComputedTorque  MotionActuationMode=InputMotion  SensePosition=off  SenseVelocity=off  SenseAcceleration=off  SenseTorqueForce=off  SenseLowerLimitTorqueForce=off  SenseUpperLimitTorqueForce=off  LowerLimitSpecify=off  LowerLimitBound=-90  LowerLimitBoundUnits=deg  LowerLimitStiffness=1e4  LowerLimitStiffnessUnits=N*m/deg  LowerLimitDamping=10  LowerLimitDampingUnits=N*m/(deg/s)  LowerLimitTransitionRegionWidth=0.1  LowerLimitTransitionRegionWidthUnits=deg  UpperLimitSpecify=off  UpperLimitBound=90  UpperLimitBoundUnits=deg  UpperLimitStiffness=1e4  UpperLimitStiffnessUnits=N*m/deg  UpperLimitDamping=10  UpperLimitDampingUnits=N*m/(deg/s)  UpperLimitTransitionRegionWidth=0.1  UpperLimitTransitionRegionWidthUnits=deg  PositionTargetSpecify=on  PositionTargetPriority=High  PositionTargetValue=0  PositionTargetValueUnits=deg  VelocityTargetSpecify=off  VelocityTargetPriority=High  VelocityTargetValue=0  VelocityTargetValueUnits=deg/s
  Rigid Transform8 : sm_lib/Frames and Transforms/Rigid Transform  TranslationMethod=None  TranslationStandardOffset=0  TranslationLengthUnit=m  TranslationStandardAxis=+Z  TranslationCartesianOffset=[0 0 0]  TranslationROffset=0  TranslationROffsetUnits=m  TranslationZOffset=0  TranslationZOffsetUnits=m  TranslationThetaOffset=0  TranslationThetaOffsetUnits=deg  RotationMethod=StandardAxis  RotationAngleUnits=deg  RotationStandardAxis=+X  RotationAngle=90  RotationArbitraryAxis=[0 0 1]  FollAlignAxisA=+X  BaseAlignAxisA=+Y  FollAlignAxisB=+Y  BaseAlignAxisB=+Z  RotationSequenceAxes=FollowerAxes  RotationSequence=XYX  RotationSequenceAngles=[0 0 0]  RotationSequenceAnglesUnits=deg  RotationMatrix=[1 0 0; 0 1 0; 0 0 1]
  Rigid Transform9 : sm_lib/Frames and Transforms/Rigid Transform  TranslationMethod=None  TranslationStandardOffset=0  TranslationLengthUnit=m  TranslationStandardAxis=+Z  TranslationCartesianOffset=[0 0 0]  TranslationROffset=0  TranslationROffsetUnits=m  TranslationZOffset=0  TranslationZOffsetUnits=m  TranslationThetaOffset=0  TranslationThetaOffsetUnits=deg  RotationMethod=StandardAxis  RotationAngleUnits=deg  RotationStandardAxis=+X  RotationAngle=90  RotationArbitraryAxis=[0 0 1]  FollAlignAxisA=+X  BaseAlignAxisA=+Y  FollAlignAxisB=+Y  BaseAlignAxisB=+Z  RotationSequenceAxes=FollowerAxes  RotationSequence=XYX  RotationSequenceAngles=[0 0 0]  RotationSequenceAnglesUnits=deg  RotationMatrix=[1 0 0; 0 1 0; 0 0 1]
  Simulink-PS Converter4 : nesl_utility/Simulink-PS Converter  PhysicalDomain=network_engine_domain  SubClassName=ps_input  LeftPortType=input  RightPortType=output  PseudoPeriodic=off  Frequencies=[]  NoiseDistribution=none  NoiseParameters=[]  Unit=1  AffineConversion=off  FilteringAndDerivatives=filter  SimscapeFilterOrder=2  InputFilterTimeConstant=0.001  UdotUserProvided=0
  B1 : PMIOPort  Side=Left
  B2 : PMIOPort  Port=2  Side=Right
  wires:
  upperJoint/1 -> Simulink-PS Converter4/1
  connections:
  Rigid Transform9/LConn1 -- B2/RConn1
  Rigid Transform8/LConn1 -- B1/RConn1
  R2/RConn1 -- Rigid Transform9/RConn1
  Rigid Transform8/RConn1 -- R2/LConn1
  Simulink-PS Converter4/RConn1 -- R2/LConn2

== system quadrupedRobot/Robot/LR/Subsystem2 ==
  lowerJoint : Inport
  R3 : sm_lib/Joints/Revolute Joint  JointMode=Normal  SenseConstraintForce=off  SenseConstraintForceX=off  SenseConstraintForceY=off  SenseConstraintForceZ=off  SenseConstraintTorque=off  SenseConstraintTorqueX=off  SenseConstraintTorqueY=off  SenseConstraintTorqueZ=off  SenseTotalForce=off  SenseTotalForceX=off  SenseTotalForceY=off  SenseTotalForceZ=off  SenseTotalTorque=off  SenseTotalTorqueX=off  SenseTotalTorqueY=off  SenseTotalTorqueZ=off  CompositeWrenchDir=FollowerOnBase  CompositeWrenchFrame=BaseFrame  EquilibriumPosition=0  EquilibriumPositionUnits=deg  SpringStiffness=0  SpringStiffnessUnits=N*m/deg  DampingCoefficient=0  DampingCoefficientUnits=N*m/(deg/s)  TorqueActuationMode=ComputedTorque  MotionActuationMode=InputMotion  SensePosition=off  SenseVelocity=off  SenseAcceleration=off  SenseTorqueForce=off  SenseLowerLimitTorqueForce=off  SenseUpperLimitTorqueForce=off  LowerLimitSpecify=off  LowerLimitBound=-90  LowerLimitBoundUnits=deg  LowerLimitStiffness=1e4  LowerLimitStiffnessUnits=N*m/deg  LowerLimitDamping=10  LowerLimitDampingUnits=N*m/(deg/s)  LowerLimitTransitionRegionWidth=0.1  LowerLimitTransitionRegionWidthUnits=deg  UpperLimitSpecify=off  UpperLimitBound=90  UpperLimitBoundUnits=deg  UpperLimitStiffness=1e4  UpperLimitStiffnessUnits=N*m/deg  UpperLimitDamping=10  UpperLimitDampingUnits=N*m/(deg/s)  UpperLimitTransitionRegionWidth=0.1  UpperLimitTransitionRegionWidthUnits=deg  PositionTargetSpecify=on  PositionTargetPriority=High  PositionTargetValue=0  PositionTargetValueUnits=deg  VelocityTargetSpecify=off  VelocityTargetPriority=High  VelocityTargetValue=0  VelocityTargetValueUnits=deg/s
  Rigid Transform8 : sm_lib/Frames and Transforms/Rigid Transform  TranslationMethod=None  TranslationStandardOffset=0  TranslationLengthUnit=m  TranslationStandardAxis=+Z  TranslationCartesianOffset=[0 0 0]  TranslationROffset=0  TranslationROffsetUnits=m  TranslationZOffset=0  TranslationZOffsetUnits=m  TranslationThetaOffset=0  TranslationThetaOffsetUnits=deg  RotationMethod=StandardAxis  RotationAngleUnits=deg  RotationStandardAxis=+X  RotationAngle=90  RotationArbitraryAxis=[0 0 1]  FollAlignAxisA=+X  BaseAlignAxisA=+Y  FollAlignAxisB=+Y  BaseAlignAxisB=+Z  RotationSequenceAxes=FollowerAxes  RotationSequence=XYX  RotationSequenceAngles=[0 0 0]  RotationSequenceAnglesUnits=deg  RotationMatrix=[1 0 0; 0 1 0; 0 0 1]
  Rigid Transform9 : sm_lib/Frames and Transforms/Rigid Transform  TranslationMethod=None  TranslationStandardOffset=0  TranslationLengthUnit=m  TranslationStandardAxis=+Z  TranslationCartesianOffset=[0 0 0]  TranslationROffset=0  TranslationROffsetUnits=m  TranslationZOffset=0  TranslationZOffsetUnits=m  TranslationThetaOffset=0  TranslationThetaOffsetUnits=deg  RotationMethod=StandardAxis  RotationAngleUnits=deg  RotationStandardAxis=+X  RotationAngle=90  RotationArbitraryAxis=[0 0 1]  FollAlignAxisA=+X  BaseAlignAxisA=+Y  FollAlignAxisB=+Y  BaseAlignAxisB=+Z  RotationSequenceAxes=FollowerAxes  RotationSequence=XYX  RotationSequenceAngles=[0 0 0]  RotationSequenceAnglesUnits=deg  RotationMatrix=[1 0 0; 0 1 0; 0 0 1]
  Simulink-PS Converter : nesl_utility/Simulink-PS Converter  PhysicalDomain=network_engine_domain  SubClassName=ps_input  LeftPortType=input  RightPortType=output  PseudoPeriodic=off  Frequencies=[]  NoiseDistribution=none  NoiseParameters=[]  Unit=1  AffineConversion=off  FilteringAndDerivatives=filter  SimscapeFilterOrder=2  InputFilterTimeConstant=0.001  UdotUserProvided=0
  B1 : PMIOPort  Side=Left
  B2 : PMIOPort  Port=2  Side=Right
  wires:
  lowerJoint/1 -> Simulink-PS Converter/1
  connections:
  Rigid Transform9/LConn1 -- B2/RConn1
  Rigid Transform8/LConn1 -- B1/RConn1
  R3/RConn1 -- Rigid Transform9/RConn1
  Simulink-PS Converter/RConn1 -- R3/LConn2
  Rigid Transform8/RConn1 -- R3/LConn1

== system quadrupedRobot/Robot/RF/LowerSys ==
  lowerJoint : Inport
  PS-Simulink Converter : nesl_utility/PS-Simulink Converter  PhysicalDomain=network_engine_domain  SubClassName=ps_output  LeftPortType=input  RightPortType=output  PseudoPeriodic=off  Frequencies=[]  Unit=inherit  AffineConversion=off
  R3 : sm_lib/Joints/Revolute Joint  JointMode=Normal  SenseConstraintForce=off  SenseConstraintForceX=off  SenseConstraintForceY=off  SenseConstraintForceZ=off  SenseConstraintTorque=off  SenseConstraintTorqueX=off  SenseConstraintTorqueY=off  SenseConstraintTorqueZ=off  SenseTotalForce=off  SenseTotalForceX=off  SenseTotalForceY=off  SenseTotalForceZ=off  SenseTotalTorque=off  SenseTotalTorqueX=off  SenseTotalTorqueY=off  SenseTotalTorqueZ=off  CompositeWrenchDir=FollowerOnBase  CompositeWrenchFrame=BaseFrame  EquilibriumPosition=0  EquilibriumPositionUnits=deg  SpringStiffness=0  SpringStiffnessUnits=N*m/deg  DampingCoefficient=0  DampingCoefficientUnits=N*m/(deg/s)  TorqueActuationMode=ComputedTorque  MotionActuationMode=InputMotion  SensePosition=off  SenseVelocity=off  SenseAcceleration=off  SenseTorqueForce=on  SenseLowerLimitTorqueForce=off  SenseUpperLimitTorqueForce=off  LowerLimitSpecify=off  LowerLimitBound=-90  LowerLimitBoundUnits=deg  LowerLimitStiffness=1e4  LowerLimitStiffnessUnits=N*m/deg  LowerLimitDamping=10  LowerLimitDampingUnits=N*m/(deg/s)  LowerLimitTransitionRegionWidth=0.1  LowerLimitTransitionRegionWidthUnits=deg  UpperLimitSpecify=off  UpperLimitBound=90  UpperLimitBoundUnits=deg  UpperLimitStiffness=1e4  UpperLimitStiffnessUnits=N*m/deg  UpperLimitDamping=10  UpperLimitDampingUnits=N*m/(deg/s)  UpperLimitTransitionRegionWidth=0.1  UpperLimitTransitionRegionWidthUnits=deg  PositionTargetSpecify=on  PositionTargetPriority=High  PositionTargetValue=0  PositionTargetValueUnits=deg  VelocityTargetSpecify=off  VelocityTargetPriority=High  VelocityTargetValue=0  VelocityTargetValueUnits=deg/s
  Rigid Transform8 : sm_lib/Frames and Transforms/Rigid Transform  TranslationMethod=None  TranslationStandardOffset=0  TranslationLengthUnit=m  TranslationStandardAxis=+Z  TranslationCartesianOffset=[0 0 0]  TranslationROffset=0  TranslationROffsetUnits=m  TranslationZOffset=0  TranslationZOffsetUnits=m  TranslationThetaOffset=0  TranslationThetaOffsetUnits=deg  RotationMethod=StandardAxis  RotationAngleUnits=deg  RotationStandardAxis=+X  RotationAngle=90  RotationArbitraryAxis=[0 0 1]  FollAlignAxisA=+X  BaseAlignAxisA=+Y  FollAlignAxisB=+Y  BaseAlignAxisB=+Z  RotationSequenceAxes=FollowerAxes  RotationSequence=XYX  RotationSequenceAngles=[0 0 0]  RotationSequenceAnglesUnits=deg  RotationMatrix=[1 0 0; 0 1 0; 0 0 1]
  Rigid Transform9 : sm_lib/Frames and Transforms/Rigid Transform  TranslationMethod=None  TranslationStandardOffset=0  TranslationLengthUnit=m  TranslationStandardAxis=+Z  TranslationCartesianOffset=[0 0 0]  TranslationROffset=0  TranslationROffsetUnits=m  TranslationZOffset=0  TranslationZOffsetUnits=m  TranslationThetaOffset=0  TranslationThetaOffsetUnits=deg  RotationMethod=StandardAxis  RotationAngleUnits=deg  RotationStandardAxis=+X  RotationAngle=90  RotationArbitraryAxis=[0 0 1]  FollAlignAxisA=+X  BaseAlignAxisA=+Y  FollAlignAxisB=+Y  BaseAlignAxisB=+Z  RotationSequenceAxes=FollowerAxes  RotationSequence=XYX  RotationSequenceAngles=[0 0 0]  RotationSequenceAnglesUnits=deg  RotationMatrix=[1 0 0; 0 1 0; 0 0 1]
  Simulink-PS Converter : nesl_utility/Simulink-PS Converter  PhysicalDomain=network_engine_domain  SubClassName=ps_input  LeftPortType=input  RightPortType=output  PseudoPeriodic=off  Frequencies=[]  NoiseDistribution=none  NoiseParameters=[]  Unit=1  AffineConversion=off  FilteringAndDerivatives=filter  SimscapeFilterOrder=2  InputFilterTimeConstant=0.001  UdotUserProvided=0
  B1 : PMIOPort  Side=Left
  B2 : PMIOPort  Port=2  Side=Right
  Torque : Outport
  wires:
  lowerJoint/1 -> Simulink-PS Converter/1
  PS-Simulink Converter/1 -> Torque/1
  connections:
  Rigid Transform9/LConn1 -- B2/RConn1
  Rigid Transform8/LConn1 -- B1/RConn1
  R3/RConn1 -- Rigid Transform9/RConn1
  Simulink-PS Converter/RConn1 -- R3/LConn2
  Rigid Transform8/RConn1 -- R3/LConn1
  PS-Simulink Converter/LConn1 -- R3/RConn2

== system quadrupedRobot/Robot/RF/ShoulderSyS ==
  shoulderJoint : Inport
  PS-Simulink Converter : nesl_utility/PS-Simulink Converter  PhysicalDomain=network_engine_domain  SubClassName=ps_output  LeftPortType=input  RightPortType=output  PseudoPeriodic=off  Frequencies=[]  Unit=inherit  AffineConversion=off
  R1 : sm_lib/Joints/Revolute Joint  JointMode=Normal  SenseConstraintForce=off  SenseConstraintForceX=off  SenseConstraintForceY=off  SenseConstraintForceZ=off  SenseConstraintTorque=off  SenseConstraintTorqueX=off  SenseConstraintTorqueY=off  SenseConstraintTorqueZ=off  SenseTotalForce=off  SenseTotalForceX=off  SenseTotalForceY=off  SenseTotalForceZ=off  SenseTotalTorque=off  SenseTotalTorqueX=off  SenseTotalTorqueY=off  SenseTotalTorqueZ=off  CompositeWrenchDir=FollowerOnBase  CompositeWrenchFrame=BaseFrame  EquilibriumPosition=0  EquilibriumPositionUnits=deg  SpringStiffness=0  SpringStiffnessUnits=N*m/deg  DampingCoefficient=0  DampingCoefficientUnits=N*m/(deg/s)  TorqueActuationMode=ComputedTorque  MotionActuationMode=InputMotion  SensePosition=off  SenseVelocity=off  SenseAcceleration=off  SenseTorqueForce=on  SenseLowerLimitTorqueForce=off  SenseUpperLimitTorqueForce=off  LowerLimitSpecify=off  LowerLimitBound=-90  LowerLimitBoundUnits=deg  LowerLimitStiffness=1e4  LowerLimitStiffnessUnits=N*m/deg  LowerLimitDamping=10  LowerLimitDampingUnits=N*m/(deg/s)  LowerLimitTransitionRegionWidth=0.1  LowerLimitTransitionRegionWidthUnits=deg  UpperLimitSpecify=off  UpperLimitBound=90  UpperLimitBoundUnits=deg  UpperLimitStiffness=1e4  UpperLimitStiffnessUnits=N*m/deg  UpperLimitDamping=10  UpperLimitDampingUnits=N*m/(deg/s)  UpperLimitTransitionRegionWidth=0.1  UpperLimitTransitionRegionWidthUnits=deg  PositionTargetSpecify=off  PositionTargetPriority=High  PositionTargetValue=0  PositionTargetValueUnits=deg  VelocityTargetSpecify=off  VelocityTargetPriority=High  VelocityTargetValue=0  VelocityTargetValueUnits=deg/s
  Rigid Transform8 : sm_lib/Frames and Transforms/Rigid Transform  TranslationMethod=None  TranslationStandardOffset=0  TranslationLengthUnit=m  TranslationStandardAxis=+Z  TranslationCartesianOffset=[0 0 0]  TranslationROffset=0  TranslationROffsetUnits=m  TranslationZOffset=0  TranslationZOffsetUnits=m  TranslationThetaOffset=0  TranslationThetaOffsetUnits=deg  RotationMethod=StandardAxis  RotationAngleUnits=deg  RotationStandardAxis=+Y  RotationAngle=90  RotationArbitraryAxis=[0 0 1]  FollAlignAxisA=+X  BaseAlignAxisA=+Y  FollAlignAxisB=+Y  BaseAlignAxisB=+Z  RotationSequenceAxes=FollowerAxes  RotationSequence=XYX  RotationSequenceAngles=[0 0 0]  RotationSequenceAnglesUnits=deg  RotationMatrix=[1 0 0; 0 1 0; 0 0 1]
  Rigid Transform9 : sm_lib/Frames and Transforms/Rigid Transform  TranslationMethod=None  TranslationStandardOffset=0  TranslationLengthUnit=m  TranslationStandardAxis=+Z  TranslationCartesianOffset=[0 0 0]  TranslationROffset=0  TranslationROffsetUnits=m  TranslationZOffset=0  TranslationZOffsetUnits=m  TranslationThetaOffset=0  TranslationThetaOffsetUnits=deg  RotationMethod=StandardAxis  RotationAngleUnits=deg  RotationStandardAxis=+Y  RotationAngle=90  RotationArbitraryAxis=[0 0 1]  FollAlignAxisA=+X  BaseAlignAxisA=+Y  FollAlignAxisB=+Y  BaseAlignAxisB=+Z  RotationSequenceAxes=FollowerAxes  RotationSequence=XYX  RotationSequenceAngles=[0 0 0]  RotationSequenceAnglesUnits=deg  RotationMatrix=[1 0 0; 0 1 0; 0 0 1]
  Simulink-PS Converter4 : nesl_utility/Simulink-PS Converter  PhysicalDomain=network_engine_domain  SubClassName=ps_input  LeftPortType=input  RightPortType=output  PseudoPeriodic=off  Frequencies=[]  NoiseDistribution=none  NoiseParameters=[]  Unit=1  AffineConversion=off  FilteringAndDerivatives=filter  SimscapeFilterOrder=2  InputFilterTimeConstant=0.001  UdotUserProvided=0
  B1 : PMIOPort  Side=Left
  B2 : PMIOPort  Port=2  Side=Right
  Torque_Shoulder : Outport
  wires:
  shoulderJoint/1 -> Simulink-PS Converter4/1
  PS-Simulink Converter/1 -> Torque_Shoulder/1
  connections:
  Rigid Transform8/RConn1 -- R1/LConn1
  Simulink-PS Converter4/RConn1 -- R1/LConn2
  R1/RConn1 -- Rigid Transform9/RConn1
  Rigid Transform8/LConn1 -- B1/RConn1
  Rigid Transform9/LConn1 -- B2/RConn1
  PS-Simulink Converter/LConn1 -- R1/RConn2
